simulink model "rotpentemplate_MPC"  (R2018b)
settings: Solver=ode45  StartTime=0.0  StopTime=30  RelTol=1e-3  EnableMultiTasking=on
InitFcn:
  | MPC
values from neighbouring files (symbols this model uses):
  h = 0.005    [LQR_main.m]    (also in Sawtooth_03_sim_validation.mat = 0.01; Sawtooth_03_sim_validationv2.mat = 0.01; Sawtooth_03_sim_validationv3.mat = 0.01; Sawtooth_03_sim_validationv4.mat = 0.01)
undefined symbols (not defined in the file or in its folder): A, adingain, adinoffs, B, daoutgain, daoutoffs, quadcost, Xref
libraries: simulink x1
settings Model: Creator=rbabuska  LastModifiedBy=janneke
settings DataIOCC: SaveFormat=Array  SignalLoggingName=sigsOut
settings OptimizationCC: BooleanDataType=off  ExpressionDepthLimit=2147483647  InitFltsAndDblsToZero=on  LifeSpan=inf
settings DebuggingCC: SaveWithParameterizedLinksMsg=none  SignalResolutionControl=TryResolveAllWithWarning  MultiTaskDSMMsg=warning  MultiTaskCondExecSysMsg=none  AllowSymbolicDim=off  StateNameClashWarn=warning  SFUnexpectedBacktrackingDiag=warning  SFNoUnconditionalDefaultTransitionDiag=warning  SFExecutionAtInitializationDiag=none
settings HardwareCC: ProdBitPerPointer=32  ProdBitPerSizeT=32  ProdBitPerPtrDiffT=32  ProdLargestAtomicFloat=None  ProdIntDivRoundTo=Undefined  ProdEndianess=Unspecified  ProdWordSize=32  ProdHWDeviceType=32-bit Generic  TargetUnknown=on
settings ModelReferenceCC: PropagateSignalLabelsOutOfModel=off
settings SFSimCC: SimUseLocalCustomCode=off
settings RTWCC: RTWUseLocalCustomCode=off
settings CodeAppCC: StateflowObjectComments=on
settings GRTTargetCC: TargetFcnLib=ansi_tfl_tmw.mat  TargetLangStandard=C89/C90 (ANSI)  GeneratePreprocessorConditionals=Disable all  CombineOutputUpdateFcns=off  GRTInterface=on
settings ConfigComp: CovMetricSettings=dw  CovHtmlReporting=on  CovSaveCumulativeToWorkspaceVar=on  CovSaveSingleToWorkspaceVar=on  CovExternalEMLEnable=off

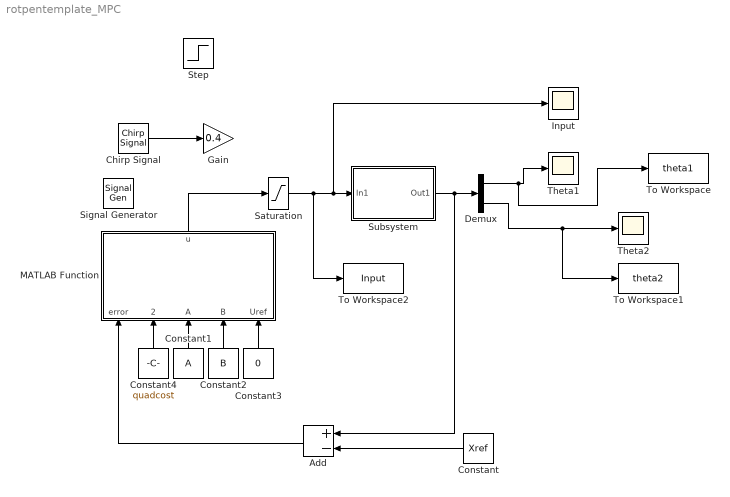
== system rotpentemplate_MPC ==
  Add : Sum  Inputs=+-
  Chirp Signal : simulink/Sources/Chirp Signal  f1=0.05  T=30  f2=1.5
  Constant : Constant  Value=Xref
  Constant1 : Constant  Value=A
  Constant2 : Constant  Value=B
  Constant3 : Constant  Value=0
  Constant4 : Constant  Value=quadcost
  Demux : Demux  Outputs=2
  Gain : Gain  Gain=0.4
  Input : Scope
  MATLAB Function : MATLAB Function  TreatAsAtomicUnit=on
  Saturation : Saturate  UpperLimit=1  LowerLimit=-1
  Signal Generator : SignalGenerator  WaveForm=square  Amplitude=0.3
  Step : Step  After=0.25  SampleTime=0
  Subsystem : Subsystem
      mask Display: disp('Rotational\nPendulum')
  Theta1 : Scope
  Theta2 : Scope
  To Workspace : ToWorkspace  VariableName=theta1  SaveFormat=Timeseries  SampleTime=-1
  To Workspace1 : ToWorkspace  VariableName=theta2  SaveFormat=Timeseries  SampleTime=-1
  To Workspace2 : ToWorkspace  VariableName=Input  SaveFormat=Timeseries  SampleTime=-1
  wires:
  Saturation/1 -> To Workspace2/1, Subsystem/1(In1), Input/1
  Subsystem/1(Out1) -> Add/1, Demux/1
  Demux/1 -> To Workspace/1, Theta1/1
  Chirp Signal/1 -> Gain/1
  Demux/2 -> To Workspace1/1, Theta2/1
  Constant/1 -> Add/2
  MATLAB Function/1(u) -> Saturation/1
  Add/1 -> MATLAB Function/1(error)
  Constant1/1 -> MATLAB Function/3(A)
  Constant2/1 -> MATLAB Function/4(B)
  Constant3/1 -> MATLAB Function/5(Uref)
  Constant4/1 -> MATLAB Function/2(quadcost)

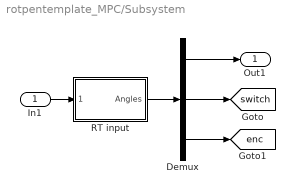
== system rotpentemplate_MPC/Subsystem ==
  In1 : Inport
  Demux : Demux  Outputs=[2 4 1]
  RT input : Subsystem  mask{Ts=h, channels=[6 7]}
      mask prompts: Ts "Sample time [s]:"; channels "Channels to read (e.g., [6 7])"
      mask init:
      | hwinit;
      | 
      | % initialize FPGA
      | fugihandle = fugiboard('Open', 'Pendulum1');
      | fugihandle.WatchdogTimeout = 0.5;
      | fugiboard('SetParams', fugihandle);
      | fugiboard('Write', fugihandle, 0, 0, 0, 0);  % dummy write to sync interface board
      | fugiboard('Write', fugihandle, 5, 1, 0, 0);  % reset position, activate relay
      | data = fugiboard('Read', fugihandle);        % get version info from FPGA
      | % model = bitshift(data(1), -5); 
      | % version = bitand(data(1), 31);
      | % disp(sprintf('FPGA setup %d, version %d', model, version)); % for the B&P it should say 1 1, or else there is a problem
      | fugiboard('Write', fugihandle, 0, 1, 0, 0);  % end reset
      | pause(0.1);                         % give relay some time to respond
      mask Display: disp('Rotational\nPendulum')
  Out1 : Outport
  tag scope: enc=global, switch=global
  wires:
  RT input/1(Angles) -> Demux/1
  Demux/1 -> Out1/1
  Demux/2 -> [switch]
  Demux/3 -> [enc]
  In1/1 -> RT input/1(Motors)

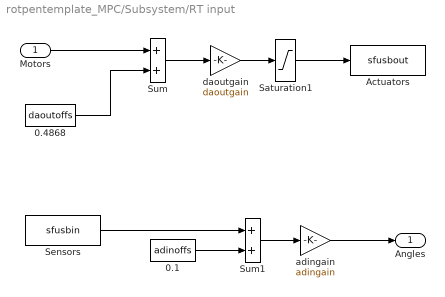
== system rotpentemplate_MPC/Subsystem/RT input ==
  Motors : Inport
  0.1 : Constant  Value=adinoffs
  0.4868 : Constant  Value=daoutoffs
  Actuators : S-Function  FunctionName=sfusbout  Parameters=Ts, fugihandle  SFunctionDeploymentMode=off  EnableBusSupport=off
  Saturation1 : Saturate  UpperLimit=10  LowerLimit=-10
  Sensors : S-Function  FunctionName=sfusbin  Parameters=Ts, fugihandle, channels  SFunctionDeploymentMode=off  EnableBusSupport=off
  Sum : Sum  SaturateOnIntegerOverflow=on  InputSameDT=on  OutDataTypeStr=Inherit: Same as first input
  Sum1 : Sum  SaturateOnIntegerOverflow=on  InputSameDT=on  OutDataTypeStr=Inherit: Same as first input
  adingain : Gain  Gain=adingain  SaturateOnIntegerOverflow=on  OutDataTypeStr=Inherit: Same as input  ParamDataTypeStr=Inherit: Same as input
  daoutgain : Gain  Gain=daoutgain  SaturateOnIntegerOverflow=on  OutDataTypeStr=Inherit: Same as input  ParamDataTypeStr=Inherit: Same as input
  Angles : Outport
  wires:
  Sum/1 -> daoutgain/1
  0.4868/1 -> Sum/2
  Motors/1 -> Sum/1
  Sum1/1 -> adingain/1
  0.1/1 -> Sum1/2
  adingain/1 -> Angles/1
  Saturation1/1 -> Actuators/1
  daoutgain/1 -> Saturation1/1
  Sensors/1 -> Sum1/1

== matlab function rotpentemplate_MPC/MATLAB Function ==
  data: error input; u output; quadcost input; A input; B input; Uref input
function u = quadprob(error,quadcost, A, B, Uref)

persistent k;
if isempty(k)
    k=1;
end
   
persistent uk;
if isempty(uk)
    uk=[0;0];
end

if k*par.Ts_b<=t   
    k=k+1;

    uB=quadprog(quadcost.H(:,:,k-1),quadcost.h(:,:,k-1)*error);
    uk=uB(1:dim.nu);
    k
    
    
end

u=uk+Uref(k,:)';
